simulink model "Zad_3_wolnozmienny"  (R2018a)
settings: Solver=FixedStepAuto  StartTime=0.0  StopTime=0  RelTol=1e-3
libraries: CPOiS_SourcesSinks x4, CPOiS_DataManipulation x2, CPOiS_General x1
settings Model: Creator=rafal  LastModifiedBy=rafal

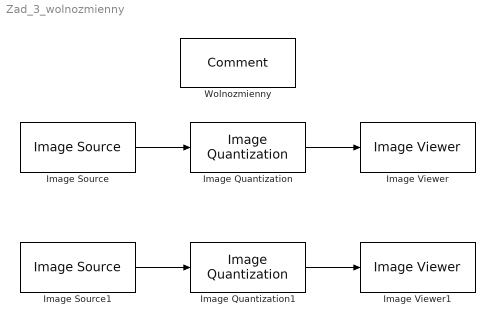
== system Zad_3_wolnozmienny ==
  Image Quantization : CPOiS_DataManipulation/Image Quantization  LevelsNum=32
      settings: SourceProductName=CPOiS - Digital image and signal processing
  Image Quantization1 : CPOiS_DataManipulation/Image Quantization  LevelsNum=8
      settings: SourceProductName=CPOiS - Digital image and signal processing
  Image Source : CPOiS_SourcesSinks/Image Source  FileSelection=ball.png
      settings: SourceProductName=CPOiS - Digital image and signal processing
  Image Source1 : CPOiS_SourcesSinks/Image Source  FileSelection=ball.png
      settings: SourceProductName=CPOiS - Digital image and signal processing
  Image Viewer : CPOiS_SourcesSinks/Image Viewer
      settings: SourceProductName=CPOiS - Digital image and signal processing
  Image Viewer1 : CPOiS_SourcesSinks/Image Viewer
      settings: SourceProductName=CPOiS - Digital image and signal processing
  "Wolnozmienny " : CPOiS_General/Comment
      settings: SourceProductName=CPOiS - Digital image and signal processing
  wires:
  Image Source/1 -> Image Quantization/1
  Image Quantization/1 -> Image Viewer/1
  Image Quantization1/1 -> Image Viewer1/1
  Image Source1/1 -> Image Quantization1/1
